simulink model "teste"  (R2023a)
settings: Solver=VariableStepAuto  StartTime=0.0  StopTime=2  RelTol=1e-3
libraries: simulink x1
settings Model: Creator=luciano  LastModifiedBy=luciano

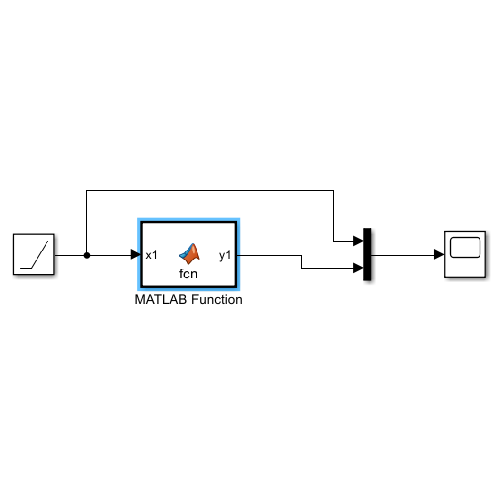
[thumbnail: Simulink's stored preview of the top-level diagram]
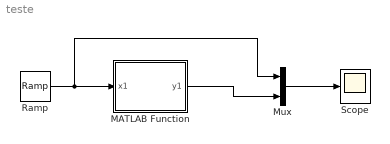
== system teste ==
  MATLAB Function : MATLAB Function  TreatAsAtomicUnit=on
  Mux : Mux  Inputs=2
  Ramp : simulink/Sources/Ramp  slope=1  start=0  InitialOutput=-1  VectorParams1D=off
  Scope : Scope
  wires:
  Ramp/1 -> Mux/1, MATLAB Function/1(x1)
  Mux/1 -> Scope/1
  MATLAB Function/1(y1) -> Mux/2

== matlab function teste/MATLAB Function ==
  data: x1 input; y1 output
function y1 = fcn(x1)
%#codegen

teste = (x1 < 0) * -1 + (x1 >= 0)
valor = x1 * teste

MIN = 0.3
valorRetorno = 0.4

v1 = (valor >= MIN) * valorRetorno
v2 = (valor < MIN) * ((valorRetorno / (MIN)) * valor)

y1 = (v1 + v2) * teste
